simulink model "Headlight_Model_New"  (R2018a)
settings: Solver=FixedStepDiscrete  StartTime=0.0  StopTime=10.0  FixedStep=1  RelTol=1e-3
undefined symbols (not defined in the file or in its folder): DN, Light, Road_T, V_Detected
libraries: simulink x20
settings Model: Creator=Shivansh  LastModifiedBy=Shivansh
settings DebuggingCC: SignalInfNanChecking=warning  UniqueDataStoreMsg=warning  StrictBusMsg=WarnOnBusTreatedAsVector

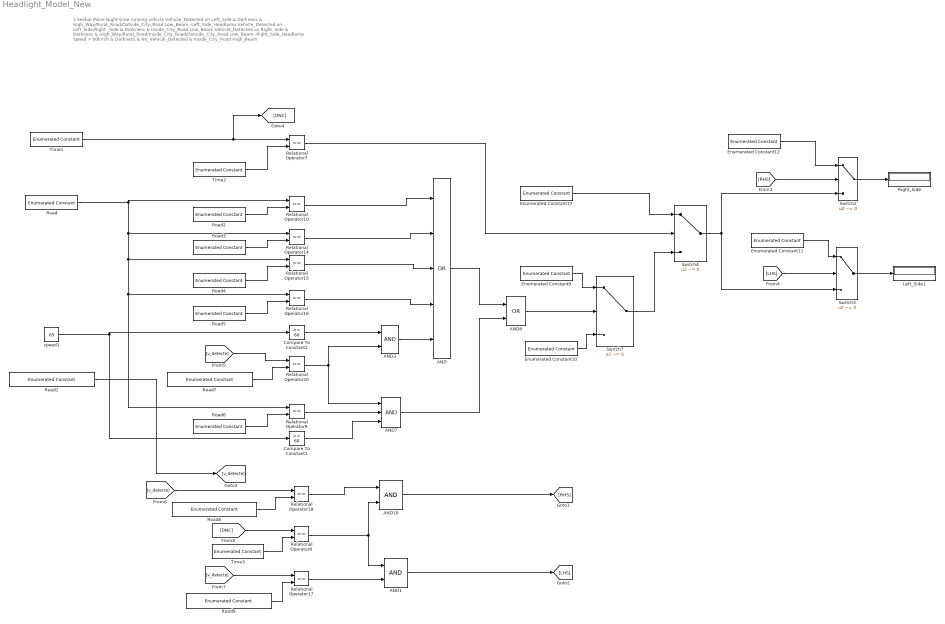
== system Headlight_Model_New ==
  note: 3
      | Snehal Mane
      | Night-time running vehicle
      | Vehicle_Detected on Left_Side & Darkness & High_Way/Rural_Road/Outside_City_Road
      | Low_Beam -Left_Side_Headlamp
      |
      | Vehicle_Detected on Left_Side/Right _Side & Darkness & Inside_City_Road
      | Low_Beam
      |
      | Vehicle_Detected on Right_Side & Darkness & High_Way/Rural_Road/Inside_City_Road/Outside_City_Road
      | Low_Beam -Right_Side_Headlamp
      |
      | Speed > 60km/h & Darkness & No_Vehical_Detected & Inside_City_Road
      | High_Beam
  AND : Logic  Operator=OR  Inputs=5  AllPortsSameDT=off  OutDataTypeStr=boolean
  AND1 : Logic  AllPortsSameDT=off  OutDataTypeStr=boolean
  AND10 : Logic  AllPortsSameDT=off  OutDataTypeStr=boolean
  AND3 : Logic  AllPortsSameDT=off  OutDataTypeStr=boolean
  AND7 : Logic  Inputs=3  AllPortsSameDT=off  OutDataTypeStr=boolean
  AND8 : Logic  Operator=OR  AllPortsSameDT=off  OutDataTypeStr=boolean
  Compare To Constant1 : simulink/Logic and Bit Operations/Compare To Constant  relop=>=  const=60  OutDataTypeStr=boolean
  Compare To Constant2 : simulink/Logic and Bit Operations/Compare To Constant  relop=>=  const=60  OutDataTypeStr=boolean
  Enumerated Constant10 : simulink/Sources/Enumerated Constant  OutDataTypeStr=Enum: Light  Value=Light.Low_Beam  SampleTime=inf
  Enumerated Constant11 : simulink/Sources/Enumerated Constant  OutDataTypeStr=Enum: Light  Value=Light.Low_Beam  SampleTime=inf
  Enumerated Constant12 : simulink/Sources/Enumerated Constant  OutDataTypeStr=Enum: Light  Value=Light.Low_Beam  SampleTime=inf
  Enumerated Constant17 : simulink/Sources/Enumerated Constant  OutDataTypeStr=Enum: Light  Value=Light.Headlight_Off  SampleTime=inf
  Enumerated Constant9 : simulink/Sources/Enumerated Constant  OutDataTypeStr=Enum: Light  Value=Light.High_beam  SampleTime=inf
  Left_Side1 : Display
  Relational Operator{7..10,14..18,20} (10 alike) : RelationalOperator  Operator===  OutDataTypeStr=boolean  RndMeth=Simplest
  Right_Side : Display
  Road : simulink/Sources/Enumerated Constant  OutDataTypeStr=Enum: Road_T  Value=Road_T.Inside_City_Road  SampleTime=inf
  Road1 : simulink/Sources/Enumerated Constant  OutDataTypeStr=Enum: V_Detected  Value=V_Detected.Vehicle_Detected_Right  SampleTime=inf
  Road2 : simulink/Sources/Enumerated Constant  OutDataTypeStr=Enum: Road_T  Value=Road_T.Express_Way  SampleTime=inf
  Road3 : simulink/Sources/Enumerated Constant  OutDataTypeStr=Enum: Road_T  Value=Road_T.High_Way  SampleTime=inf
  Road4 : simulink/Sources/Enumerated Constant  OutDataTypeStr=Enum: Road_T  Value=Road_T.Rural_Road  SampleTime=inf
  Road5 : simulink/Sources/Enumerated Constant  OutDataTypeStr=Enum: Road_T  Value=Road_T.Outside_City_Road  SampleTime=inf
  Road6 : simulink/Sources/Enumerated Constant  OutDataTypeStr=Enum: Road_T  Value=Road_T.Inside_City_Road  SampleTime=inf
  Road7 : simulink/Sources/Enumerated Constant  OutDataTypeStr=Enum: V_Detected  Value=V_Detected.No_Vehical_Detected  SampleTime=inf
  Road8 : simulink/Sources/Enumerated Constant  OutDataTypeStr=Enum: V_Detected  Value=V_Detected.Vehicle_Detected_Right  SampleTime=inf
  Road9 : simulink/Sources/Enumerated Constant  OutDataTypeStr=Enum: V_Detected  Value=V_Detected.Vehicle_Detected_Left  SampleTime=inf
  Switch{2..4,7} (4 alike) : Switch  Criteria=u2 ~= 0
  Time1 : simulink/Sources/Enumerated Constant  OutDataTypeStr=Enum: DN  Value=DN.Darkness  SampleTime=inf
  Time2 : simulink/Sources/Enumerated Constant  OutDataTypeStr=Enum: DN  Value=DN.Day_Time  SampleTime=inf
  Time3 : simulink/Sources/Enumerated Constant  OutDataTypeStr=Enum: DN  Value=DN.Darkness  SampleTime=inf
  speed1 : Constant  Value=65
  wires:
  Switch3/1 -> Left_Side1/1
  Enumerated Constant12/1 -> Switch2/1
  Time2/1 -> Relational Operator7/2
  Relational Operator17/1 -> AND1/2
  Relational Operator16/1 -> AND/4
  [DNC] -> Relational Operator8/1
  Enumerated Constant11/1 -> Switch3/1
  speed1/1 -> Compare To Constant1/1, Compare To Constant2/1
  Road1/1 -> [v_detecte]
  AND1/1 -> [LHS]
  [v_detecte] -> Relational Operator20/1
  Relational Operator20/1 -> AND7/1, AND3/2
  Switch4/1 -> Switch2/3, Switch3/3
  Road4/1 -> Relational Operator15/2
  Relational Operator8/1 -> AND1/1, AND10/2
  Relational Operator7/1 -> Switch4/2
  Enumerated Constant10/1 -> Switch7/3
  Road8/1 -> Relational Operator18/2
  Road3/1 -> Relational Operator14/2
  Compare To Constant2/1 -> AND3/1
  Road/1 -> Relational Operator10/1, Relational Operator9/1, Relational Operator16/1, Relational Operator15/1, Relational Operator14/1
  Enumerated Constant17/1 -> Switch4/1
  AND3/1 -> AND/5
  Road9/1 -> Relational Operator17/2
  Switch2/1 -> Right_Side/1
  AND/1 -> AND8/1
  [v_detecte] -> Relational Operator17/1
  Enumerated Constant9/1 -> Switch7/1
  Switch7/1 -> Switch4/3
  Compare To Constant1/1 -> AND7/3
  Relational Operator10/1 -> AND/1
  Road2/1 -> Relational Operator10/2
  Relational Operator15/1 -> AND/3
  AND7/1 -> AND8/2
  AND10/1 -> [RHS]
  Relational Operator14/1 -> AND/2
  Road5/1 -> Relational Operator16/2
  Relational Operator18/1 -> AND10/1
  Relational Operator9/1 -> AND7/2
  [LHS] -> Switch3/2
  [v_detecte] -> Relational Operator18/1
  Time1/1 -> [DNC], Relational Operator7/1
  [RHS] -> Switch2/2
  AND8/1 -> Switch7/2
  Road7/1 -> Relational Operator20/2
  Road6/1 -> Relational Operator9/2
  Time3/1 -> Relational Operator8/2
